simulink model "alalalt"  (R2021b)
settings: Solver=VariableStepAuto  StartTime=0.0  StopTime=10.0  RelTol=1e-3
settings Model: Creator=Voic  LastModifiedBy=Voic

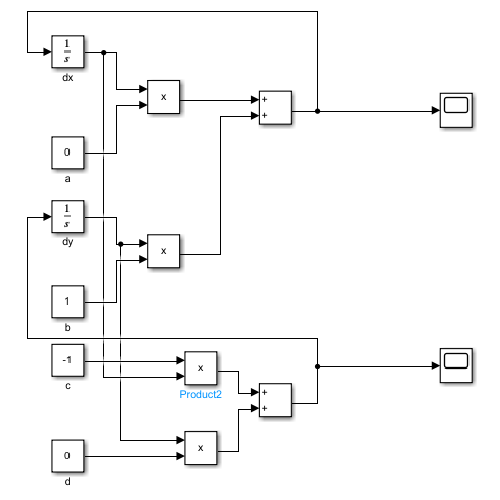
[thumbnail: Simulink's stored preview of the top-level diagram]
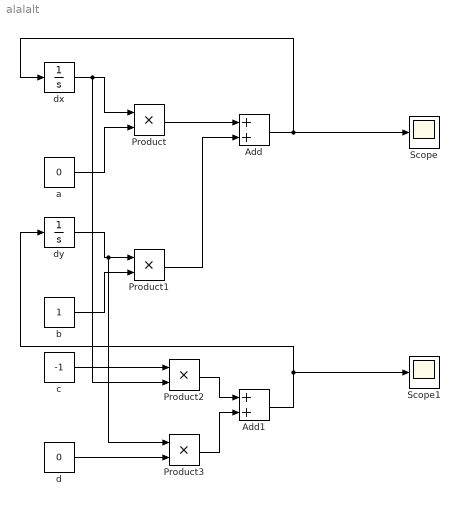
== system alalalt ==
  Add : Sum
  Add1 : Sum
  Product{,1..3} (4 alike) : Product
  Scope : Scope
  Scope1 : Scope
  a : Constant  Value=0
  b : Constant
  c : Constant  Value=-1
  d : Constant  Value=0
  dx : Integrator  InitialCondition=1
  dy : Integrator  InitialCondition=2
  wires:
  dx/1 -> Product2/2, Product/1
  a/1 -> Product/2
  Product/1 -> Add/1
  dy/1 -> Product3/1, Product1/1
  b/1 -> Product1/2
  Product1/1 -> Add/2
  Add/1 -> Scope/1, dx/1
  Product2/1 -> Add1/1
  Product3/1 -> Add1/2
  Add1/1 -> Scope1/1, dy/1
  c/1 -> Product2/1
  d/1 -> Product3/2
